simulink model "DSB_SC_mixing_diode_demod_2020"  (R2021a)
settings: Solver=VariableStepAuto  StartTime=0.0  StopTime=0.2  RelTol=1e-3
PreLoadFcn:
  | Df = 0;
values from neighbouring files (symbols this model uses):
  seed = input('Enter your student ID: ')    [DSBAMsignals.m]    (also in DSBAMsignals_rand.m; DSB_SC_sinusoidals.m)
libraries: dsparch4 x1
settings Model: Creator=14083  LastModifiedBy=000098944
settings SolverCC: AlgebraicLoopSolver=TrustRegion
settings DebuggingCC: SFMachineParentedDataDiag=warning

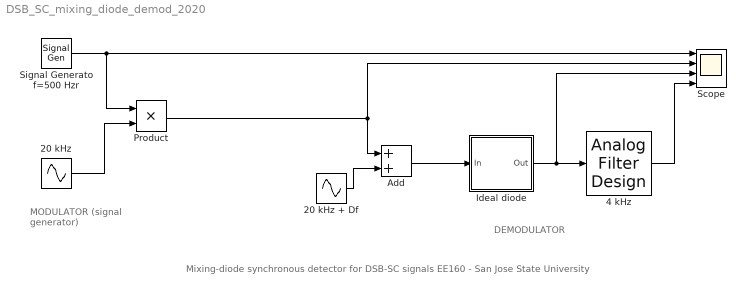
== system DSB_SC_mixing_diode_demod_2020 ==
  note: Mixing-diode synchronous detector for DSB-SC signals
      | EE160 - San Jose State University
  note: DEMODULATOR
  note: MODULATOR
      | (signal generator)
  20 kHz : Sin  Frequency=2*pi*20000  Samples=3  SampleTime=(1/20000)/10  VectorParams1D=off
  20 kHz + Df : Sin  Amplitude=2+0.75*mod(seed,11)/11  Frequency=2*pi*20000+Df  Samples=3  SampleTime=(1/20000)/10  VectorParams1D=off
  4 kHz : dsparch4/Analog Filter Design  method=Butterworth  filttype=Lowpass  N=4  Wlo=2*pi*5000  Whi=80  Rp=0.001  Rs=80
  Add : Sum
  Ideal diode : Subsystem  TreatAsAtomicUnit=on
  Product : Product
  Scope : Scope  NumInputPorts=4
  Signal Generato f=500 Hzr : SignalGenerator  Frequency=500
  wires:
  20 kHz/1 -> Product/2
  Product/1 -> Scope/2, Add/1
  Ideal diode/1(Out) -> Scope/3, 4 kHz/1
  Signal Generato f=500 Hzr/1 -> Product/1, Scope/1
  20 kHz + Df/1 -> Add/2
  Add/1 -> Ideal diode/1(In)
  4 kHz/1 -> Scope/4

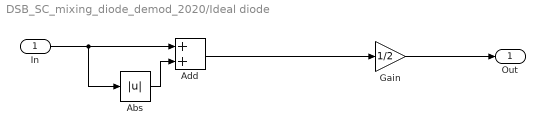
== system DSB_SC_mixing_diode_demod_2020/Ideal diode ==
  In : Inport
  Abs : Abs
  Add : Sum
  Gain : Gain  Gain=1/2
  Out : Outport
  wires:
  Add/1 -> Gain/1
  Abs/1 -> Add/2
  In/1 -> Abs/1, Add/1
  Gain/1 -> Out/1
